simulink model "BLDC_OpenLoop_s32k144"  (Simulink 9.0)
settings: Solver=FixedStepDiscrete  StartTime=0.0  StopTime=10.0  FixedStep=0.1  RelTol=1e-3  EnableMultiTasking=on
InitFcn:
  | mbd_s32k_consistency_checks(bdroot(gcs));
undefined symbols (not defined in the file): External, LQFP, One, Shot, TRGMUX_PDB_TRIG
libraries: mbd_s32k1xx_ec_toolbox x40, simulink x8, mbd_msd_ec_toolbox x5, ammclib_bam_s32k14x x2
(part 2 of 2)

== system BLDC_OpenLoop_s32k144/S32K144 EVB/Trapezoidal_Control/SixStepCommutationLogic/Do_Alignment/CW Dir ==
  Action Port : ActionPort  ActionPortLabel=if((u1 >= 0))
  Constant : Constant  Value=2  OutDataTypeStr=Inherit: Inherit via back propagation
  Constant1 : Constant  Value=0  OutDataTypeStr=Inherit: Inherit via back propagation
  Constant2 : Constant  OutDataTypeStr=Inherit: Inherit via back propagation
  Out1 : Outport
  Out2 : Outport  Port=2
  Out3 : Outport  Port=3
  wires:
  Constant/1 -> Out1/1
  Constant2/1 -> Out3/1
  Constant1/1 -> Out2/1

== stateflow chart S32K144 EVB/Trapezoidal_Control/SixStepCommutationLogic/Alignment_Counter/Align Sequence ==
  settings: sampleTime=0.500
  (default) -> (junction 7)
  (junction 7) -> (junction 8) [order 1] : [DelayTimeIn > ALIGN_TIME]
      | {ExecuteAlign = 0;}
  (junction 7) -> (junction 9) [order 2]
  (junction 8) -> (junction 10)
  (junction 9) -> (junction 10) : {DelayTimeOut = DelayTimeIn + 1;
      | ExecuteAlign = 1;}
  data: DelayTimeOut output uint16; DelayTimeIn input uint16; ExecuteAlign output boolean; ALIGN_TIME parameter double

== stateflow chart S32K144 EVB/Control_Logic/Enable PDB and start FTM ==
  settings: sampleTime=0.500
  state END
  state A
  (default) -> A
  A -> END : /*Post initializations*/
      | {enablePDB;}
  END -> END : {Normal_Op;}
  events: enablePDB output FUNCTION_CALL_EVENT; Normal_Op output FUNCTION_CALL_EVENT

== stateflow chart S32K144 EVB/Event_Control/ControlPollingLogic ==
  state Logic1
    Logic1 -> (junction 28)
    (default) -> (junction 28)
    (junction 28) -> (junction 29) [order 1] : [(VoltageChange <= V0) && (VoltageChange >= -V0)]
        | {Trigger;}
    (junction 28) -> (junction 30) [order 2]
    (junction 29) -> (junction 31)
    (junction 30) -> (junction 31)
  (default) -> Logic1
  data: VoltageChange input single; V0 parameter double
  events: Trigger output FUNCTION_CALL_EVENT

== stateflow chart S32K144 EVB/IO Controls /If Action Subsystem/Chart ==
  state SwitchCheck1 [parallel]
    settings: executionOrder=1
    state Decrement
      du:out = 0;
      (default) -> (junction 50)
      Decrement -> (junction 50) [order 1] : [((Increment ==0)& ...
          |  (Decrement==1))& hasChanged(Increment)]
          | {out=-0.1;}
    state Increment
      du:out = 0;
      (default) -> (junction 53)
      Increment -> (junction 53) [order 1] : [((Increment ==1)& ...
          |  (Decrement==0))&hasChanged(Decrement)]
          | {out=0.1;}
    (default) -> Decrement : { out =0;}
    Increment -> Decrement [order 1] : [(Increment==0)& ...
        |  (Decrement==1) ...
        | & hasChanged(Increment)]
        | {out=-0.1;}
    Decrement -> Increment [order 1] : [((Increment ==1)& ...
        |  (Decrement==0))&hasChanged(Decrement)]
        | {out=0.1;}
  data: out output single; Increment input boolean; Decrement input boolean

== stateflow chart S32K144 EVB/Trapezoidal_Control/SixStepCommutationLogic/Normal_Run/CommutationTableLookup ==
  (default) -> (junction 68)
  (junction 68) -> (junction 69) [order 1] : /*CCW*/
      | [DIR < 0]
  (junction 68) -> (junction 70) [order 2] : /*CW*/
      | [DIR >= 0]
  (junction 69) -> (junction 71) : {
      |    Phase_A = ccwTable[HALL_STATE][0];
      |    Phase_B = ccwTable[HALL_STATE][1];
      |    Phase_C = ccwTable[HALL_STATE][2];
      | }
  (junction 70) -> (junction 71) : {
      |    Phase_A = cwTable[HALL_STATE][0];
      |    Phase_B = cwTable[HALL_STATE][1];
      |    Phase_C = cwTable[HALL_STATE][2];
      | }
  data: ccwTable constant uint8 size=[8 3] =[0 0 0; 0 2 1; 2 1 0; 2 0 1; 1 0 2; 1 2 0; 0 1 2; 0 0 0;]; HALL_STATE input uint8; Phase_A output uint8; Phase_B output uint8; Phase_C output uint8; cwTable constant uint8 size=[8 3] =[0 0 0; 0 1 2; 1 2 0; 1 0 2; 2 0 1; 2 1 0; 0 2 1; 0 0 0;]; DIR input int16

== stateflow chart S32K144 EVB/Trapezoidal_Control/PhaseSwitchLogic ==
  settings: sampleTime=0.500
  note: Phase States:
      | 0 = NC
      | 1 = -Vdcb
      | 2 = +Vdcb
  (default) -> (junction 90)
  (junction 90) -> (junction 91) [order 1] : /*check for phase state 0 */
      | [Phase_A == 0]
      | /*set output for state 0 */
      | {Phase_A_HS = 0; Phase_A_LS =0;}
  (junction 90) -> (junction 92) [order 2]
  (junction 91) -> (junction 93)
  (junction 92) -> (junction 93) [order 1] : /*check for phase state 1 */
      | [Phase_A == 1]
      | /*set output for state 1 */
      | {Phase_A_HS = 0; Phase_A_LS = PWM_Duty_Cycle;}
  (junction 92) -> (junction 94) [order 2]
  (junction 93) -> (junction 95)
  (junction 94) -> (junction 95) [order 1] : /*check for phase state 2 */
      | [Phase_A == 2]
      | /*set output for state 2 */
      | {Phase_A_HS = 1; Phase_A_LS = 0;}
  (junction 94) -> (junction 96) [order 2]
  (junction 95) -> (junction 97)
  (junction 96) -> (junction 97)
  (junction 97) -> (junction 98) [order 1] : /*check for phase state 0 */
      | [Phase_B == 0]
      | /*set output for state 0 */
      | {Phase_B_HS = 0; Phase_B_LS = 0;}
  (junction 97) -> (junction 99) [order 2]
  (junction 98) -> (junction 100)
  (junction 99) -> (junction 100) [order 1] : /*check for phase state 1 */
      | [Phase_B == 1]
      | /*set output for state 1 */
      | {Phase_B_HS = 0; Phase_B_LS = PWM_Duty_Cycle;}
  (junction 99) -> (junction 101) [order 2]
  (junction 100) -> (junction 102)
  (junction 101) -> (junction 102) [order 1] : /*check for phase state 2 */
      | [Phase_B == 2]
      | /*set output for state 2 */
      | {Phase_B_HS = 1; Phase_B_LS = 0;}
  (junction 101) -> (junction 103) [order 2]
  (junction 102) -> (junction 104)
  (junction 103) -> (junction 104)
  (junction 104) -> (junction 105) [order 1] : /*check for phase state 0 */
      | [Phase_C == 0]
      | /*set output for state 0 */
      | {Phase_C_HS = 0; Phase_C_LS = 0;}
  (junction 104) -> (junction 106) [order 2]
  (junction 105) -> (junction 107)
  (junction 106) -> (junction 107) [order 1] : /*check for phase state 1 */
      | [Phase_C == 1]
      | /*set output for state 1 */
      | {Phase_C_HS = 0; Phase_C_LS = PWM_Duty_Cycle;}
  (junction 106) -> (junction 108) [order 2]
  (junction 107) -> (junction 109)
  (junction 108) -> (junction 109) [order 1] : /*check for phase state 2 */
      | [Phase_C == 2]
      | /*set output for state 2 */
      | {Phase_C_HS = 1; Phase_C_LS = 0;}
  (junction 108) -> (junction 110) [order 2]
  (junction 109) -> (junction 111)
  (junction 110) -> (junction 111)
  data: Phase_A input double; Phase_B input double; Phase_C input double; Phase_A_HS output single; Phase_A_LS output single; Phase_B_HS output single; Phase_B_LS output single; Phase_C_HS output single; Phase_C_LS output single; PWM_Duty_Cycle input single

== stateflow chart S32K144 EVB/Event_Control/Init ==
  settings: sampleTime=0.500
  state A
  state B
  (default) -> A
  A -> B : {Init;
      | index=0;}
  data: index local double
  events: Init output FUNCTION_CALL_EVENT
